simulink model "driving_dynamics_model"  (R2023a)
settings: Solver=VariableStepAuto  StartTime=0.0  StopTime=10.0  RelTol=1e-3
values from neighbouring files (symbols this model uses):
  a = 1.8    [longitudinal_driving_parameters.m]
  A = 1.25    [longitudinal_driving_parameters.m]
  a1R = -1e-5    (= -1e-05)    [longitudinal_driving_parameters.m]
  a2R = 1.25    [longitudinal_driving_parameters.m]
  BR = 5.7507    [longitudinal_driving_parameters.m]
  cd = 0.4    [longitudinal_driving_parameters.m]
  CR = 1.2421    [longitudinal_driving_parameters.m]
  cz = 1    [longitudinal_driving_parameters.m]
  enginemap = [-0.15, 0.23, 0.60, 0.68, 0.8 ... (first row only)    [longitudinal_driving_parameters.m]
  enginerpm = linspace(1000,15000,15)'    [longitudinal_driving_parameters.m]
  ER = -6.8251    [longitudinal_driving_parameters.m]
  g = 9.81    [longitudinal_driving_parameters.m]
  h = 0.2    [longitudinal_driving_parameters.m]
  i_initial = 5    [longitudinal_driving_parameters.m]
  igear = [23.10, 17.64, 13.86, 10.92, 8.82, 7.13, 5.88, 4.33]'    [longitudinal_driving_parameters.m]
  Iwheel = 0.9    [longitudinal_driving_parameters.m]
  L = 3.5    [longitudinal_driving_parameters.m]
  m = 850    [longitudinal_driving_parameters.m]
  r = 0.375    [longitudinal_driving_parameters.m]
  rho = 1.225    [longitudinal_driving_parameters.m]
  rpm_idling = 1000    [longitudinal_driving_parameters.m]
  rpm_limit = 15000    [longitudinal_driving_parameters.m]
  rpm_up = 13500    [longitudinal_driving_parameters.m]
  Tengmax = 250    [longitudinal_driving_parameters.m]
  throttlepos = [0, 0.25, 0.5, 0.75, 1]'    [longitudinal_driving_parameters.m]
  TPS = 1    [longitudinal_driving_parameters.m]
  V0 = 120    [longitudinal_driving_parameters.m]
settings Model: Creator=Cassio.Freitas  LastModifiedBy=Cassio de Freitas
settings SolverCC: AlgebraicLoopSolver=TrustRegion
settings DataIOCC: ReturnWorkspaceOutputs=off
settings DebuggingCC: UnconnectedInputMsg=warning  UnconnectedOutputMsg=warning  UnconnectedLineMsg=warning  ArithmeticOperatorsInVariantConditions=warning
settings ModelReferenceCC: EnableRefExpFcnMdlSchedulingChecks=on
settings SFSimCC: CustomCodeUndefinedFunction=UseInterfaceOnly

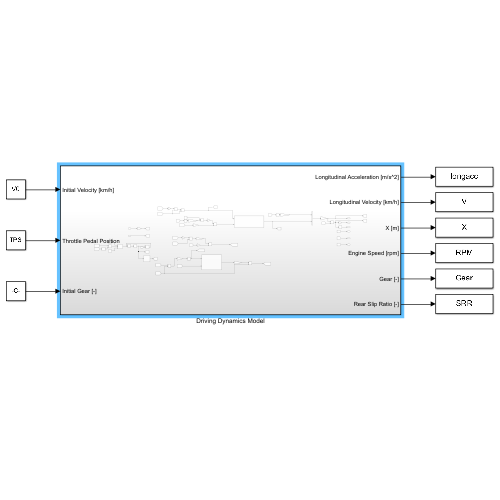
[thumbnail: Simulink's stored preview of the top-level diagram]
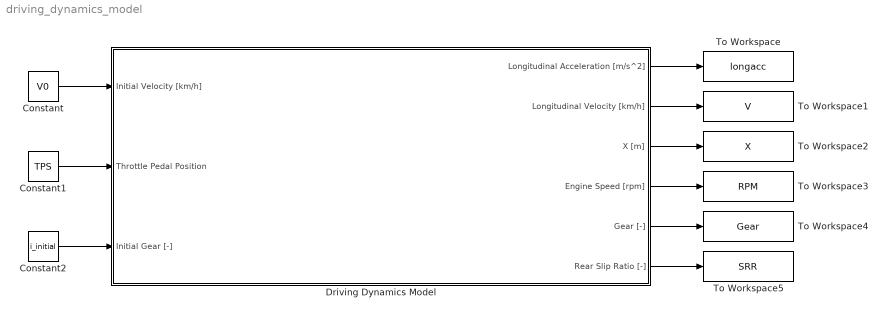
== system driving_dynamics_model ==
  Constant : Constant  Value=V0
  Constant1 : Constant  Value=TPS
  Constant2 : Constant  Value=i_initial
  "Driving Dynamics Model " : Subsystem
  To Workspace : ToWorkspace  VariableName=longacc  SaveFormat=Timeseries  SampleTime=-1
  To Workspace1 : ToWorkspace  VariableName=V  SaveFormat=Timeseries  SampleTime=-1
  To Workspace2 : ToWorkspace  VariableName=X  SaveFormat=Timeseries  SampleTime=-1
  To Workspace3 : ToWorkspace  VariableName=RPM  SaveFormat=Timeseries  SampleTime=-1
  To Workspace4 : ToWorkspace  VariableName=Gear  SaveFormat=Timeseries  SampleTime=-1
  To Workspace5 : ToWorkspace  VariableName=SRR  SaveFormat=Timeseries  SampleTime=-1
  wires:
  Constant/1 -> "Driving Dynamics Model "/1(Initial Velocity [km/h])
  Constant1/1 -> "Driving Dynamics Model "/2(Throttle Pedal Position)
  Constant2/1 -> "Driving Dynamics Model "/3(Initial Gear [-])
  "Driving Dynamics Model "/1(Longitudinal Acceleration [m/s^2]) -> To Workspace/1
  "Driving Dynamics Model "/2(Longitudinal Velocity [km/h]) -> To Workspace1/1
  "Driving Dynamics Model "/3(X [m]) -> To Workspace2/1
  "Driving Dynamics Model "/4(Engine Speed [rpm]) -> To Workspace3/1
  "Driving Dynamics Model "/5(Gear [-]) -> To Workspace4/1
  "Driving Dynamics Model "/6(Rear Slip Ratio [-]) -> To Workspace5/1

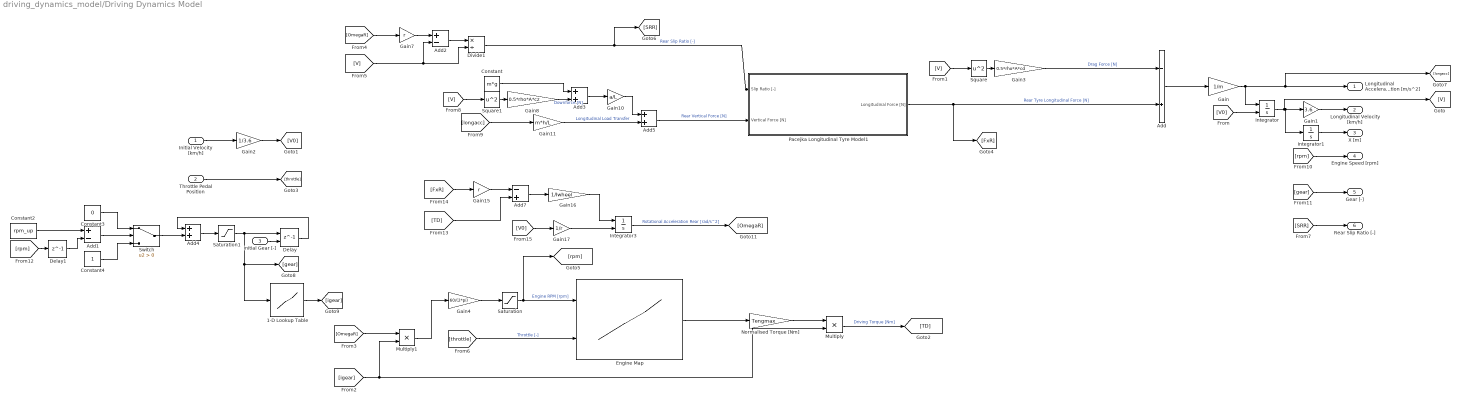
== system driving_dynamics_model/Driving Dynamics Model  ==
  Initial Velocity [km/h] : Inport
  Throttle Pedal Position : Inport  Port=2
  Initial Gear [-] : Inport  Port=3
  1-D Lookup Table : Lookup_n-D  NumberOfTableDimensions=1  BreakpointsForDimension1=[1:8]  Table=igear  InternalRulePriority=Speed  RndMeth=Simplest
  Add : Sum  Inputs=-+
  Add1 : Sum  Inputs=+-
  Add2 : Sum  Inputs=+-
  Add3 : Sum
  Add4 : Sum
  Add5 : Sum
  Add7 : Sum  Inputs=-+
  Constant : Constant  Value=m*g
  Constant2 : Constant  Value=rpm_up
  Constant3 : Constant  Value=0
  Constant4 : Constant
  Delay : Delay  DelayLength=1  InitialConditionSource=Input port
      settings: InputPortMap=u0,p4
  Delay1 : Delay  DelayLength=1
  Divide1 : Product  Inputs=*/
  Engine Map : Lookup_n-D  BreakpointsForDimension1=enginerpm  BreakpointsForDimension2=throttlepos  Table=enginemap  InternalRulePriority=Speed  RndMeth=Simplest
      settings: InputPortMap=u0,u1
  Gain : Gain  Gain=1/m
  Gain1 : Gain  Gain=3.6
  Gain10 : Gain  Gain=a/L
  Gain11 : Gain  Gain=m*h/L
  Gain15 : Gain  Gain=r
  Gain16 : Gain  Gain=1/Iwheel
  Gain17 : Gain  Gain=1/r
  Gain2 : Gain  Gain=1/3.6
  Gain3 : Gain  Gain=0.5*rho*A*cd
  Gain4 : Gain  Gain=60/(2*pi)
  Gain7 : Gain  Gain=r
  Gain8 : Gain  Gain=0.5*rho*A*cz
  Integrator : Integrator  InitialConditionSource=external
  Integrator1 : Integrator
  Integrator3 : Integrator  InitialConditionSource=external
  Multiply : Product
  Multiply1 : Product
  "Normalised Torque [Nm] " : Gain  Gain=Tengmax
  Pacejka Longitudinal Tyre Model1 : Subsystem
  Saturation : Saturate  UpperLimit=rpm_limit  LowerLimit=rpm_idling
  Saturation1 : Saturate  UpperLimit=8  LowerLimit=1
  Square : Math  Operator=square  SignedPower=on
  Square1 : Math  Operator=square  SignedPower=on
  Switch : Switch  Criteria=u2 > Threshold  SaturateOnIntegerOverflow=off  InputSameDT=off
  Longitudinal Acceleration [m/s^2] : Outport  VectorParamsAs1DForOutWhenUnconnected=off
  Longitudinal Velocity [km/h] : Outport  Port=2  VectorParamsAs1DForOutWhenUnconnected=off
  X [m] : Outport  Port=3  VectorParamsAs1DForOutWhenUnconnected=off
  Engine Speed [rpm] : Outport  Port=4  VectorParamsAs1DForOutWhenUnconnected=off
  Gear [-] : Outport  Port=5  VectorParamsAs1DForOutWhenUnconnected=off
  Rear Slip Ratio [-] : Outport  Port=6  VectorParamsAs1DForOutWhenUnconnected=off
  wires:
  Gain3/1 -> Add/1  "Drag Force [N]"
  [longacc] -> Gain11/1
  Gain17/1 -> Integrator3/2
  Gain8/1 -> Add3/2  "Downforce [N]"
  Gain2/1 -> [V0]
  Throttle Pedal Position/1 -> [throttle]
  [V] -> Square/1
  Gain15/1 -> Add7/1
  Square/1 -> Gain3/1
  [V] -> Square1/1
  [FxR] -> Gain15/1
  Add7/1 -> Gain16/1
  Add5/1 -> Pacejka Longitudinal Tyre Model1/2(Vertical Force [N])  "Rear Vertical Force [N]"
  Integrator3/1 -> [OmegaR]  "Rotational Acceleration Rear [rad/s^2]"
  [V0] -> Gain17/1
  Add/1 -> Gain/1
  Initial Velocity [km/h]/1 -> Gain2/1
  [OmegaR] -> Gain7/1
  Divide1/1 -> [SRR], Pacejka Longitudinal Tyre Model1/1(Slip Ratio [-])  "Rear Slip Ratio [-]"
  Constant/1 -> Add3/1
  Gain11/1 -> Add5/2  "Longitudinal Load Transfer"
  Integrator1/1 -> X [m]/1
  Pacejka Longitudinal Tyre Model1/1(Longitudinal Force [N]) -> Add/2, [FxR]  "Rear Tyre Longitudinal Force [N]"
  Add3/1 -> Gain10/1
  Integrator/1 -> [V], Integrator1/1, Gain1/1
  Gain7/1 -> Add2/1
  Add2/1 -> Divide1/1
  Square1/1 -> Gain8/1
  [V] -> Add2/2, Divide1/2
  Gain16/1 -> Integrator3/1
  Gain1/1 -> Longitudinal Velocity [km/h]/1
  [TD] -> Add7/2
  [V0] -> Integrator/2
  Gain/1 -> Integrator/1, [longacc], Longitudinal Acceleration [m/s^2]/1
  [SRR] -> Rear Slip Ratio [-]/1
  Gain10/1 -> Add5/1
  "Normalised Torque [Nm] "/1 -> Multiply/1
  [igear] -> Multiply1/2, Multiply/2
  Multiply/1 -> [TD]  "Driving Torque [Nm]"
  Engine Map/1 -> "Normalised Torque [Nm] "/1
  [throttle] -> Engine Map/2  "Throttle [-]"
  [OmegaR] -> Multiply1/1
  Gain4/1 -> Saturation/1
  Multiply1/1 -> Gain4/1
  [rpm] -> Engine Speed [rpm]/1
  [gear] -> Gear [-]/1
  Saturation/1 -> [rpm], Engine Map/1  "Engine RPM [rpm]"
  Constant2/1 -> Add1/1
  [rpm] -> Delay1/1
  Add1/1 -> Switch/2
  Constant3/1 -> Switch/1
  Constant4/1 -> Switch/3
  Initial Gear [-]/1 -> Delay/2
  Add4/1 -> Saturation1/1
  Delay/1 -> Add4/1
  Delay1/1 -> Add1/2
  Switch/1 -> Add4/2
  1-D Lookup Table/1 -> [igear]
  Saturation1/1 -> 1-D Lookup Table/1, [gear], Delay/1

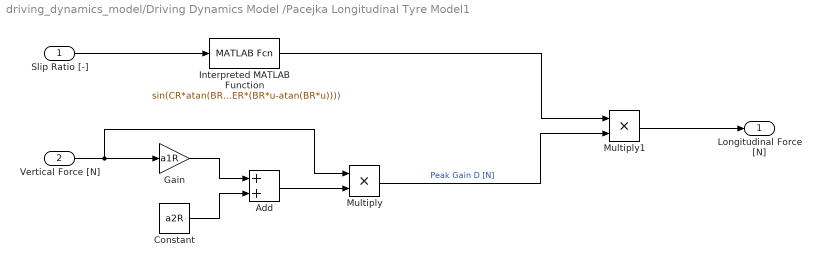
== system driving_dynamics_model/Driving Dynamics Model /Pacejka Longitudinal Tyre Model1 ==
  Slip Ratio [-] : Inport
  Vertical Force [N] : Inport  Port=2
  Add : Sum
  Constant : Constant  Value=a2R
  Gain : Gain  Gain=a1R
  Interpreted MATLAB Function : MATLABFcn  MATLABFcn=sin(CR*atan(BR*u-ER*(BR*u-atan(BR*u))))
  Multiply : Product
  Multiply1 : Product
  Longitudinal Force [N] : Outport  VectorParamsAs1DForOutWhenUnconnected=off
  wires:
  Vertical Force [N]/1 -> Multiply/1, Gain/1
  Constant/1 -> Add/2
  Gain/1 -> Add/1
  Add/1 -> Multiply/2
  Multiply/1 -> Multiply1/2  "Peak Gain D [N]"
  Slip Ratio [-]/1 -> Interpreted MATLAB Function/1
  Interpreted MATLAB Function/1 -> Multiply1/1
  Multiply1/1 -> Longitudinal Force [N]/1
